simulink model "power_arcmodels"  (Simulink 6.0)
settings: Solver=ode23tb  StartTime=0.0  StopTime=.04  RelTol=1e-5  AbsTol=1.e-5
libraries: powerlib x26
settings Model: Creator=dkennedy  LastModifiedBy=batserve  ExtModeTrigMode=oneshot  ExtModeArmWhenConnect=off  ExtModeAutoUpdateStatusClock=off
settings DataIOCC: LimitDataPoints=off  SignalLoggingName=sigsOut
settings OptimizationCC: BlockReduction=off  BooleanDataType=off
settings DebuggingCC: AlgebraicLoopMsg=none  SolverPrmCheckMsg=none
settings HardwareCC: TargetUnknown=on

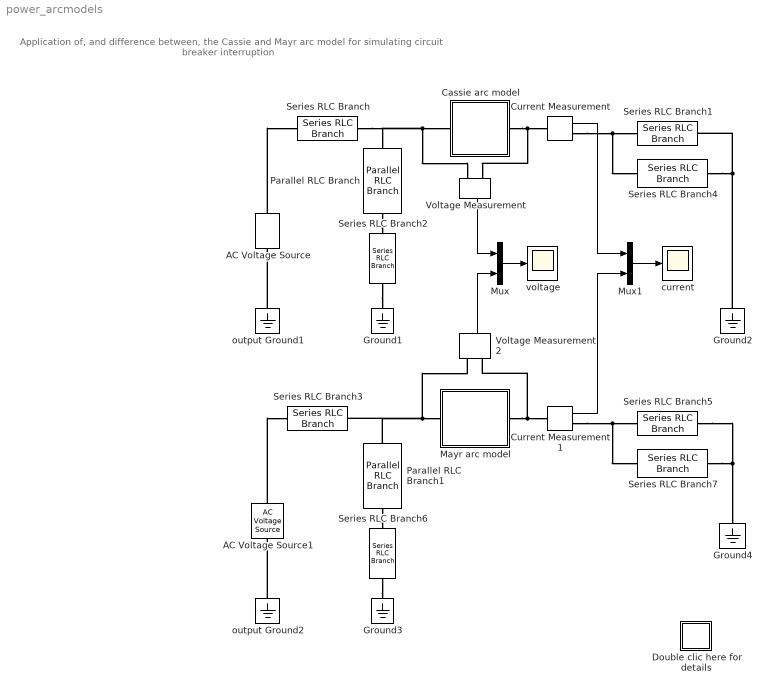
== system power_arcmodels ==
  note: Application of, and difference between, the Cassie and Mayr arc model
      | for simulating circuit breaker interruption
  AC Voltage Source : powerlib/Electrical Sources/AC Voltage Source  Description=source block  Orientation=up  Amplitude=59196  Phase=90  Frequency=60  SampleTime=0  Measurements=None
      settings: AttributesFormatString=\n
  AC Voltage Source1 : powerlib/Electrical Sources/AC Voltage Source  Description=source block  Orientation=up  Amplitude=59196  Phase=90  Frequency=60  SampleTime=0  Measurements=None
      settings: AttributesFormatString=\n
  Cassie arc model : Subsystem  AncestorBlock=arc_model/Cassie arc model  mask(Cassie arc model){tau=1.2e-6, Uc=3850, x0=1.e4, cb_trip=.02}
      mask prompts: tau "tau [s]"; Uc "Uc [V]"; x0 "g(0) [S]"; cb_trip "circuit breaker contact separation starts at [s]"
      mask help: The Cassie arc model with a constant time parameter tau and a constant arc voltage Uc: dlng/dt=1/tau*((u^2/Uc^2)-1.
      mask Help:
      | The Cassie arc model with a constant time parameter tau and a constant arc voltage Uc: dlng/dt=1/tau*((u^2/Uc^2)-1.
      | 
      | The initial conductance of the arc g(0) can be altered. Furthermore, the time at which the contact separation of the circuit breaker takes place can be specified. Until that time the arc model behaves as a conductance with the value g(0).
      mask Display: plot(-15,10,115,90,[-15,15],[50,50],[85,115],[50,50],[15,15,25,25,15],[55,45,45,55,55],[75,75,85,85,75],[55,45,45,55,55],[25,75],[50,70])
  Current Measurement : powerlib/Measurements/Current Measurement  Tag=PoWeRsYsTeMmEaSuReMeNt  PhasorSimulation=off  OutputType=Magnitude  PSBequivalent=0
  Current Measurement1 : powerlib/Measurements/Current Measurement  Tag=PoWeRsYsTeMmEaSuReMeNt  PhasorSimulation=off  OutputType=Magnitude  PSBequivalent=0
  Double clic here for details : Subsystem
      mask Display: disp('?')
  Ground{1..4} (4 alike) : powerlib/Elements/Ground  Orientation=down  PhysicalDomain=powersysdomain  SubClassName=unknown  LeftPortType=p1  RightPortType=p1  LConnTagsString=a
  Mayr arc model : Subsystem  AncestorBlock=arc_model/Mayr arc model  mask(Mayr arc model){tau=0.3e-6, P=30900, x0=1.e4, cb_trip=.02}
      mask prompts: tau "tau [s]"; P "P [W]"; x0 "g(0) [S]"; cb_trip "circuit breaker contact separation starts at [s]"
      mask help: The Mayr arc model with a constant time parameter tau and constant cooling power P: dlng/dt=1/tau*((ui/P)-1).
      mask Help:
      | The Mayr arc model with a constant time parameter tau and constant cooling power P: dlng/dt=1/tau*((ui/P)-1).
      | 
      | The initial conductance of the arc g(0) can be altered. Furthermore, the time at which the contact separation of the circuit breaker takes place can be specified. Until that time the arc model behaves as a conductance with the value g(0).
      mask Display: plot(-15,10,115,90,[-15,15],[50,50],[85,115],[50,50],[15,15,25,25,15],[55,45,45,55,55],[75,75,85,85,75],[55,45,45,55,55],[25,75],[50,70])
  Mux : Mux  Inputs=2
  Mux1 : Mux  Inputs=2
  Parallel RLC Branch : powerlib/Elements/Parallel RLC Branch  Orientation=down  PhysicalDomain=powersysdomain  SubClassName=unknown  LeftPortType=p1  RightPortType=p1  LConnTagsString=a  RConnTagsString=__new0  Resistance=29.8  Inductance=5.28e-3  Capacitance=0  Measurements=None
  Parallel RLC Branch1 : powerlib/Elements/Parallel RLC Branch  Orientation=down  PhysicalDomain=powersysdomain  SubClassName=unknown  LeftPortType=p1  RightPortType=p1  LConnTagsString=a  RConnTagsString=__new0  Resistance=29.8  Inductance=5.28e-3  Capacitance=0  Measurements=None
  Series RLC Branch : powerlib/Elements/Series RLC Branch  PhysicalDomain=powersysdomain  SubClassName=unknown  LeftPortType=p1  RightPortType=p1  LConnTagsString=__new0  RConnTagsString=__new0  Resistance=0  Inductance=3.52e-03  Capacitance=inf  Measurements=None
  Series RLC Branch1 : powerlib/Elements/Series RLC Branch  PhysicalDomain=powersysdomain  SubClassName=unknown  LeftPortType=p1  RightPortType=p1  LConnTagsString=__new0  RConnTagsString=__new0  Resistance=0  Inductance=6.256e-4  Capacitance=inf  Measurements=None
  Series RLC Branch2 : powerlib/Elements/Series RLC Branch  Orientation=down  PhysicalDomain=powersysdomain  SubClassName=unknown  LeftPortType=p1  RightPortType=p1  LConnTagsString=__new0  RConnTagsString=__new0  Resistance=0  Inductance=0  Capacitance=1.98e-6  Measurements=None
  Series RLC Branch3 : powerlib/Elements/Series RLC Branch  PhysicalDomain=powersysdomain  SubClassName=unknown  LeftPortType=p1  RightPortType=p1  LConnTagsString=__new0  RConnTagsString=__new0  Resistance=0  Inductance=3.52e-03  Capacitance=inf  Measurements=None
  Series RLC Branch4 : powerlib/Elements/Series RLC Branch  PhysicalDomain=powersysdomain  SubClassName=unknown  LeftPortType=p1  RightPortType=p1  LConnTagsString=__new0  RConnTagsString=__new0  Resistance=450  Inductance=0  Capacitance=1.93e-9  Measurements=None
  Series RLC Branch5 : powerlib/Elements/Series RLC Branch  PhysicalDomain=powersysdomain  SubClassName=unknown  LeftPortType=p1  RightPortType=p1  LConnTagsString=__new0  RConnTagsString=__new0  Resistance=0  Inductance=6.256e-4  Capacitance=inf  Measurements=None
  Series RLC Branch6 : powerlib/Elements/Series RLC Branch  Orientation=down  PhysicalDomain=powersysdomain  SubClassName=unknown  LeftPortType=p1  RightPortType=p1  LConnTagsString=__new0  RConnTagsString=__new0  Resistance=0  Inductance=0  Capacitance=1.98e-6  Measurements=None
  Series RLC Branch7 : powerlib/Elements/Series RLC Branch  PhysicalDomain=powersysdomain  SubClassName=unknown  LeftPortType=p1  RightPortType=p1  LConnTagsString=__new0  RConnTagsString=__new0  Resistance=450  Inductance=0  Capacitance=1.93e-9  Measurements=None
  Voltage Measurement : powerlib/Measurements/Voltage Measurement  Tag=PoWeRsYsTeMmEaSuReMeNt  Orientation=down  PhasorSimulation=off  OutputType=Magnitude  PSBequivalent=0
  Voltage Measurement2 : powerlib/Measurements/Voltage Measurement  Tag=PoWeRsYsTeMmEaSuReMeNt  Orientation=up  PhasorSimulation=off  OutputType=Magnitude  PSBequivalent=0
  current : Scope
      settings: TimeRange=0.04  YMin=-40000  YMax=40000
  output Ground1 : powerlib/Elements/Ground  Orientation=down  PhysicalDomain=powersysdomain  SubClassName=unknown  LeftPortType=p1  RightPortType=p1  LConnTagsString=a
  output Ground2 : powerlib/Elements/Ground  Orientation=down  PhysicalDomain=powersysdomain  SubClassName=unknown  LeftPortType=p1  RightPortType=p1  LConnTagsString=a
  voltage : Scope
      settings: TimeRange=0.04  YMin=-100000  YMax=60000
  wires:
  Mux/1 -> voltage/1
  Mux1/1 -> current/1
  Voltage Measurement/1 -> Mux/1
  Voltage Measurement2/1 -> Mux/2
  Current Measurement/1 -> Mux1/1
  Current Measurement1/1 -> Mux1/2
  connections:
  output Ground1/LConn1 -- AC Voltage Source/LConn1
  Parallel RLC Branch/RConn1 -- Series RLC Branch2/LConn1
  Series RLC Branch2/RConn1 -- Ground1/LConn1
  AC Voltage Source/RConn1 -- Series RLC Branch/LConn1
  Series RLC Branch/RConn1 -- Parallel RLC Branch/LConn1 -- Cassie arc model/LConn1 -- Voltage Measurement/LConn1
  Current Measurement/RConn1 -- Series RLC Branch1/LConn1 -- Series RLC Branch4/LConn1
  Ground2/LConn1 -- Series RLC Branch1/RConn1 -- Series RLC Branch4/RConn1
  Cassie arc model/RConn1 -- Voltage Measurement/LConn2 -- Current Measurement/LConn1
  output Ground2/LConn1 -- AC Voltage Source1/LConn1
  Parallel RLC Branch1/RConn1 -- Series RLC Branch6/LConn1
  Series RLC Branch6/RConn1 -- Ground3/LConn1
  AC Voltage Source1/RConn1 -- Series RLC Branch3/LConn1
  Parallel RLC Branch1/LConn1 -- Series RLC Branch3/RConn1 -- Mayr arc model/LConn1 -- Voltage Measurement2/LConn1
  Current Measurement1/RConn1 -- Series RLC Branch5/LConn1 -- Series RLC Branch7/LConn1
  Series RLC Branch5/RConn1 -- Ground4/LConn1 -- Series RLC Branch7/RConn1
  Mayr arc model/RConn1 -- Current Measurement1/LConn1 -- Voltage Measurement2/LConn2

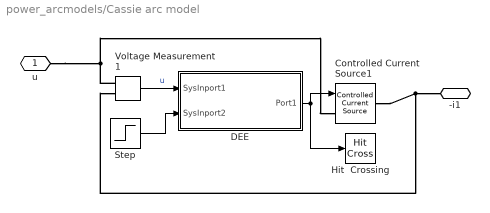
== system power_arcmodels/Cassie arc model ==
  Controlled Current Source1 : powerlib/Electrical Sources/Controlled Current Source  Description=source block  Initialize=on  Amplitude=0  Phase=0  Frequency=0  Measurements=None
      settings: AttributesFormatString=\n
  DEE : Subsystem
      settings: OpenFcn=diffeqed
      mask Type: Differential Equation Editor (DEE)
      mask Display: disp('Cassie arc model')
  Hit  Crossing : HitCross  ZeroCross=off  ShowOutputPort=off
  Step : Step  Time=cb_trip  SampleTime=0  ZeroCross=off
  Voltage Measurement1 : powerlib/Measurements/Voltage Measurement  Tag=PoWeRsYsTeMmEaSuReMeNt  PhasorSimulation=off  OutputType=Magnitude  PSBequivalent=0
  u : PMIOPort  Port=1  Side=Left
  -i1 : PMIOPort  Orientation=left  Port=2  Side=Right
  wires:
  Step/1 -> DEE/2(SysInport2)
  DEE/1(Port1) -> Hit  Crossing/1, Controlled Current Source1/1
  Voltage Measurement1/1 -> DEE/1(SysInport1)  "u"
  connections:
  Controlled Current Source1/RConn1 -- -i1/RConn1 -- Voltage Measurement1/LConn2
  Voltage Measurement1/LConn1 -- Controlled Current Source1/LConn1 -- u/RConn1

== system power_arcmodels/Double clic here for details ==
  note: Two identical circuits are displayed: one with a Cassie and one with a Mayr arc model.
      | The circuit is a simple representation of a circuit breaker interrupting a short-line fault.
      | At the source side of the circuit breaker a circuit is present for reproducing a (2-parameter
      | IEC) transient recovery voltage, while the RLC circuit at the line side represents a short
      | transmission line that is short circuited.
      |
      | A stiff solver is recommended for this type of problems due to the nonlinear
      | behaviour of the arc.
  note: This demonstration illustrates use of the Cassie and Mayr arc model
      | for simulating high voltage circuit breaker interruption
  note: Demonstration
  note: Circuit Description
  note: A blockset containing 7 arc models can be downloaded freely from the following website of the
      | Power Systems Laboratory of the Delft University of Technology: http://eps.et.tudelft.nl
      | A PDF manual with installation instructions, arc model descriptions and references to relevant
      | literature is included.
  note: Arc Model Blockset at http://eps.et.tudelft.nl
  note: The circuit breaker interruption can be started by means of the 'Start/Pause Simulation' button.
      | The voltages over both the Cassie (yellow) and Mayr arc model are displayed in one scope.
      | The currents through both the Cassie (yellow) and Mayr arc model are displayed in one scope.
      |
      | The following observations become clear from the simulation:
      | The arc behaves as a non-linear resistance; therefore both arc current and voltage pass
      | the zero value at the same time. As the power input into the arc channel is zero
      | at that time, the current zero crossing is the place where the interruption takes
      | place.
      |
      | The Cassie arc model has a constant arc voltage in the high current interval, while the
      | Mayr arc model shows an increasing arc voltage (the extinction peak) close to the
      | current zero crossing.
      |
      | The Cassie arc model fails to interrupt the short circuit current, while the Mayr arc model
      | interrupts and shows a small post-arc current of 0.6A immediately after the current zero
      | crossing. This current is caused by the transient recovery voltage building up over the
      | non-infinite arc resistance.
      |
      | In case of the Mayr arc model (the successfull interruption), the transient recovery voltage
      | (TRV) builds up over the breaker. This voltage consists of the 2-parameter TRV and the high
      | frequency voltage oscillation of the line side, which you can observe by zooming in.
  note: P.H. Schavemaker, Power Systems Laboratory,
      | Delft University of Technology, the Netherlands
      |
      | P.H.Schavemaker@its.tudelft.nl

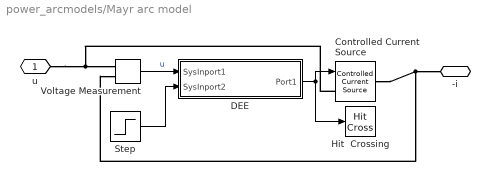
== system power_arcmodels/Mayr arc model ==
  Controlled Current Source : powerlib/Electrical Sources/Controlled Current Source  Description=source block  Initialize=on  Amplitude=0  Phase=0  Frequency=0  Measurements=None
      settings: AttributesFormatString=\n
  DEE : Subsystem
      settings: OpenFcn=diffeqed
      mask Type: Differential Equation Editor (DEE)
      mask Display: disp('Mayr arc model')
  Hit  Crossing : HitCross  ZeroCross=off  ShowOutputPort=off
  Step : Step  Time=cb_trip  SampleTime=0  ZeroCross=off
  Voltage Measurement : powerlib/Measurements/Voltage Measurement  Tag=PoWeRsYsTeMmEaSuReMeNt  PhasorSimulation=off  OutputType=Magnitude  PSBequivalent=0
  u : PMIOPort  Port=1  Side=Left
  -i : PMIOPort  Orientation=left  Port=2  Side=Right
  wires:
  Step/1 -> DEE/2(SysInport2)
  DEE/1(Port1) -> Hit  Crossing/1, Controlled Current Source/1
  Voltage Measurement/1 -> DEE/1(SysInport1)  "u"
  connections:
  Controlled Current Source/RConn1 -- Voltage Measurement/LConn2 -- -i/RConn1
  Controlled Current Source/LConn1 -- Voltage Measurement/LConn1 -- u/RConn1

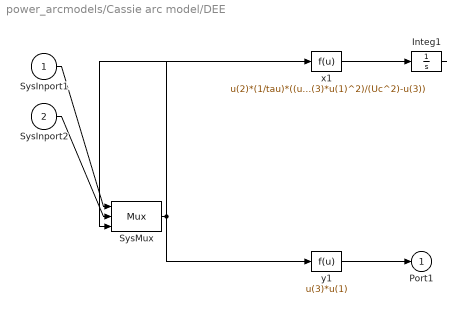
== system power_arcmodels/Cassie arc model/DEE ==
  SysInport1 : Inport  Port=1  LatchInput=off
  SysInport2 : Inport  Port=2  LatchInput=off
  Integ1 : Integrator  InitialCondition=x0  ZeroCross=off
  SysMux : Mux  Inputs=3
  x1 : Fcn  Expr=u(2)*(1/tau)*((u(3)*u(1)^2)/(Uc^2)-u(3))
  y1 : Fcn  Expr=u(3)*u(1)
  Port1 : Outport  InitialOutput=0
  wires:
  SysInport1/1 -> SysMux/1
  SysInport2/1 -> SysMux/2
  SysMux/1 -> x1/1, y1/1
  x1/1 -> Integ1/1
  Integ1/1 -> SysMux/3
  y1/1 -> Port1/1

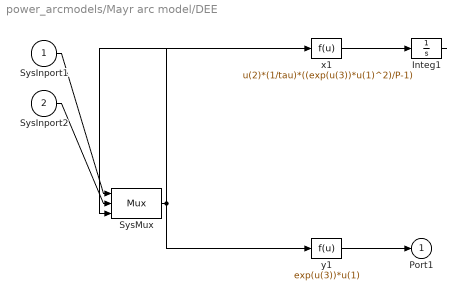
== system power_arcmodels/Mayr arc model/DEE ==
  SysInport1 : Inport  Port=1  LatchInput=off
  SysInport2 : Inport  Port=2  LatchInput=off
  Integ1 : Integrator  InitialCondition=log(x0)  ZeroCross=off
  SysMux : Mux  Inputs=3
  x1 : Fcn  Expr=u(2)*(1/tau)*((exp(u(3))*u(1)^2)/P-1)
  y1 : Fcn  Expr=exp(u(3))*u(1)
  Port1 : Outport  InitialOutput=0
  wires:
  y1/1 -> Port1/1
  SysMux/1 -> y1/1, x1/1
  Integ1/1 -> SysMux/3
  x1/1 -> Integ1/1
  SysInport2/1 -> SysMux/2
  SysInport1/1 -> SysMux/1
